simulink model "all_basic_operations"  (R2024b)
settings: Solver=ode3  StartTime=0.0  StopTime=10.0  FixedStep=0.01  RelTol=1e-3
libraries: simulink x2
settings Model: Creator=balaj  LastModifiedBy=balaj

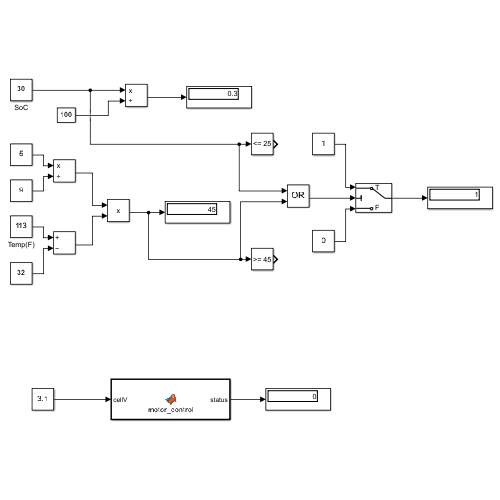
[thumbnail: Simulink's stored preview of the top-level diagram]
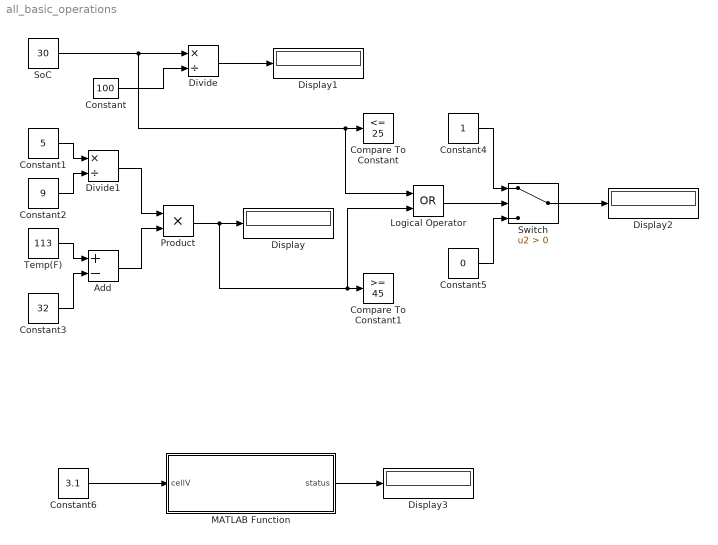
== system all_basic_operations ==
  Add : Sum  Inputs=+-
  Compare To Constant : simulink/Logic and Bit Operations/Compare To Constant  relop=<=  const=25  OutDataTypeStr=boolean
  Compare To Constant1 : simulink/Logic and Bit Operations/Compare To Constant  relop=>=  const=45  OutDataTypeStr=boolean
  Constant : Constant  Value=100
  Constant1 : Constant  Value=5
  Constant2 : Constant  Value=9
  Constant3 : Constant  Value=32
  Constant4 : Constant
  Constant5 : Constant  Value=0
  Constant6 : Constant  Value=3.1
  Display{,1..3} (4 alike) : Display
  Divide : Product  Inputs=*/
  Divide1 : Product  Inputs=*/
  Logical Operator : Logic  Operator=OR  AllPortsSameDT=off  OutDataTypeStr=boolean
  MATLAB Function : MATLAB Function  TreatAsAtomicUnit=on
  Product : Product
  SoC : Constant  Value=30
  Switch : Switch  Criteria=u2 > Threshold  SaturateOnIntegerOverflow=off  InputSameDT=off
  Temp(F) : Constant  Value=113
  wires:
  SoC/1 -> Logical Operator/1, Compare To Constant/1, Divide/1
  Constant/1 -> Divide/2
  Constant1/1 -> Divide1/1
  Constant2/1 -> Divide1/2
  Temp(F)/1 -> Add/1
  Constant3/1 -> Add/2
  Divide1/1 -> Product/1
  Add/1 -> Product/2
  Product/1 -> Logical Operator/2, Compare To Constant1/1, Display/1
  Divide/1 -> Display1/1
  Logical Operator/1 -> Switch/2
  Constant4/1 -> Switch/1
  Constant5/1 -> Switch/3
  Switch/1 -> Display2/1
  Constant6/1 -> MATLAB Function/1(cellV)
  MATLAB Function/1(status) -> Display3/1

== matlab function all_basic_operations/MATLAB Function ==
  data: cellV input; status output
function status = motor_control(cellV)
    if cellV < 3.2
        disp('Undervoltage Lockout: Motor Disabled');
        status = 0;
    else
        disp('Normal voltage Lockout: Motor Enabled');
        status = 1;
    end
end
